simulink model "magnet_field"  (R2023b)
settings: Solver=VariableStepAuto  StartTime=0.0  StopTime=10.0  RelTol=1e-3
values from neighbouring files (symbols this model uses):
  A1 = importdata("igrfSg.txt")    [SAD_project_code.m]
  A2 = importdata("igrfSh.txt")    [SAD_project_code.m]
  n_earth = sqrt(mu_E/a^3)    [SAD_project_code.m]
  timeoflaunch = date2mjd2000(date0)    [SAD_project_code.m]
libraries: simulink_extras x3
settings Model: Creator=edoardonicolucci  LastModifiedBy=edoardonicolucci

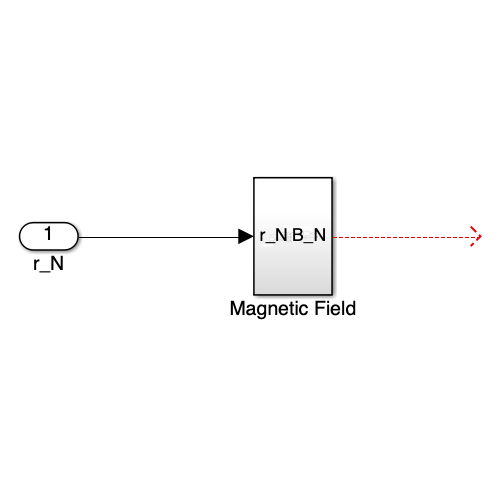
[thumbnail: Simulink's stored preview of the top-level diagram]
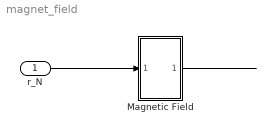
== system magnet_field ==
  r_N : Inport
  Magnetic Field : Subsystem
  wires:
  r_N/1 -> Magnetic Field/1(r_N)
  Magnetic Field/1(B_N) -> ?

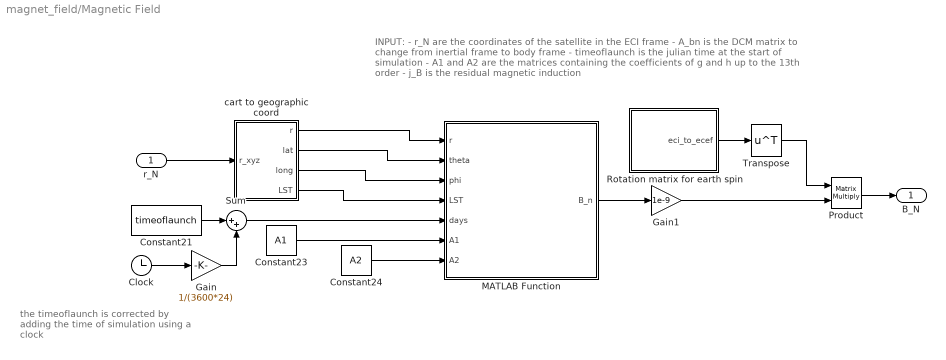
== system magnet_field/Magnetic Field ==
  note: INPUT:
      | - r_N are the coordinates of the satellite in the ECI frame
      | - A_bn is the DCM matrix to change from inertial frame to body frame
      | - timeoflaunch is the julian time at the start of simulation
      | - A1 and A2 are the matrices containing the coefficients of g and h up to the 13th order
      | - j_B is the residual magnetic induction
  note: the timeoflaunch is corrected by adding the time of simulation using a clock
  r_N : Inport
  Clock : Clock
  Constant21 : Constant  Value=timeoflaunch
  Constant23 : Constant  Value=A1
  Constant24 : Constant  Value=A2
  Gain : Gain  Gain=1/(3600*24)
  Gain1 : Gain  Gain=1e-9
  MATLAB Function : MATLAB Function  TreatAsAtomicUnit=on
  Product : Product  Multiplication=Matrix(*)
  Rotation matrix for earth spin : Subsystem
  Sum : Sum  Inputs=|++
  Transpose : Math  Operator=transpose
  cart to geographic coord : Subsystem
  B_N : Outport
  wires:
  Gain/1 -> Sum/2
  Constant23/1 -> MATLAB Function/6(A1)
  Constant24/1 -> MATLAB Function/7(A2)
  Product/1 -> B_N/1
  Constant21/1 -> Sum/1
  MATLAB Function/1(B_n) -> Gain1/1
  cart to geographic coord/4(LST) -> MATLAB Function/4(LST)
  r_N/1 -> cart to geographic coord/1(r_xyz)
  Rotation matrix for earth spin/1(eci_to_ecef) -> Transpose/1
  cart to geographic coord/2(lat) -> MATLAB Function/2(theta)
  Clock/1 -> Gain/1
  Transpose/1 -> Product/1
  cart to geographic coord/3(long) -> MATLAB Function/3(phi)
  Sum/1 -> MATLAB Function/5(days)
  cart to geographic coord/1(r) -> MATLAB Function/1(r)
  Gain1/1 -> Product/2

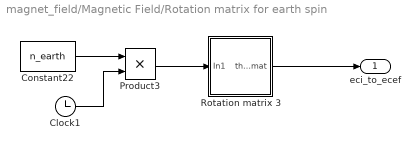
== system magnet_field/Magnetic Field/Rotation matrix for earth spin ==
  Clock1 : Clock
  Constant22 : Constant  Value=n_earth
  Product3 : Product
  Rotation matrix 3 : Subsystem
  eci_to_ecef : Outport
  wires:
  Rotation matrix 3/1(theta_mat) -> eci_to_ecef/1
  Product3/1 -> Rotation matrix 3/1(In1)
  Constant22/1 -> Product3/1
  Clock1/1 -> Product3/2

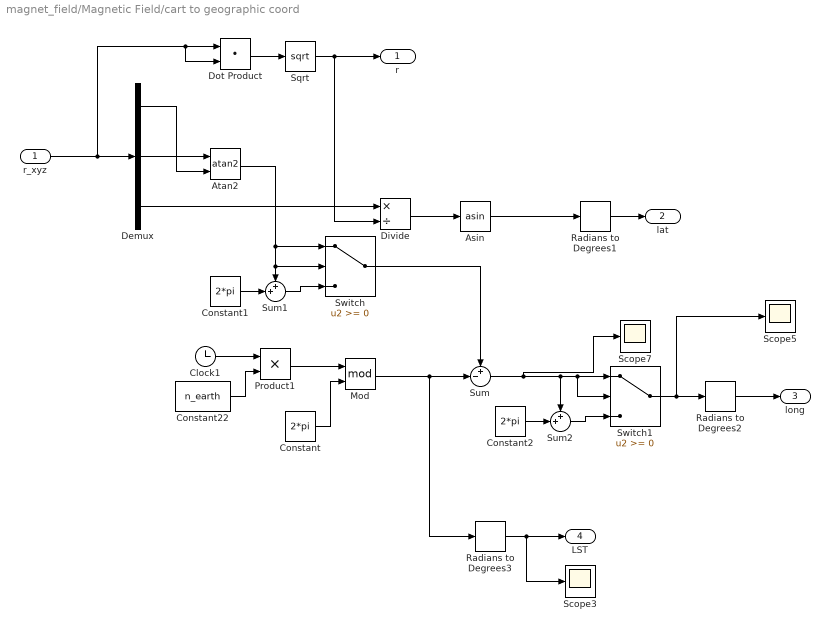
== system magnet_field/Magnetic Field/cart to geographic coord ==
  r_xyz : Inport
  Asin : Trigonometry  Operator=asin
  Atan2 : Trigonometry  Operator=atan2
  Clock1 : Clock
  Constant : Constant  Value=2*pi
  Constant1 : Constant  Value=2*pi
  Constant2 : Constant  Value=2*pi
  Constant22 : Constant  Value=n_earth
  Demux : Demux  Outputs=3
  Divide : Product  Inputs=*/
  Dot Product : DotProduct  OutDataTypeStr=Inherit: Inherit via internal rule
  Mod : Math  Operator=mod
  Product1 : Product
  Radians to Degrees1 : simulink_extras/Transformations/Radians to Degrees
  Radians to Degrees2 : simulink_extras/Transformations/Radians to Degrees
  Radians to Degrees3 : simulink_extras/Transformations/Radians to Degrees
  Scope3 : Scope
  Scope5 : Scope
  Scope7 : Scope
  Sqrt : Sqrt
  Sum : Sum  Inputs=+-|
  Sum1 : Sum  Inputs=++|
  Sum2 : Sum  Inputs=++|
  Switch : Switch  SaturateOnIntegerOverflow=off  InputSameDT=off
  Switch1 : Switch  SaturateOnIntegerOverflow=off  InputSameDT=off
  r : Outport
  lat : Outport  Port=2
  long : Outport  Port=3
  LST : Outport  Port=4
  wires:
  r_xyz/1 -> Dot Product/2, Dot Product/1, Demux/1
  Asin/1 -> Radians to Degrees1/1
  Dot Product/1 -> Sqrt/1
  Sqrt/1 -> r/1, Divide/2
  Demux/3 -> Divide/1
  Divide/1 -> Asin/1
  Demux/2 -> Atan2/1
  Demux/1 -> Atan2/2
  Constant22/1 -> Product1/2
  Clock1/1 -> Product1/1
  Sum/1 -> Scope7/1, Sum2/1, Switch1/2, Switch1/1
  Radians to Degrees3/1 -> Scope3/1, LST/1
  Mod/1 -> Radians to Degrees3/1, Sum/2
  Constant/1 -> Mod/2
  Atan2/1 -> Switch/1, Sum1/1, Switch/2
  Sum1/1 -> Switch/3
  Constant1/1 -> Sum1/2
  Sum2/1 -> Switch1/3
  Constant2/1 -> Sum2/2
  Switch1/1 -> Scope5/1, Radians to Degrees2/1
  Switch/1 -> Sum/1
  Radians to Degrees1/1 -> lat/1
  Radians to Degrees2/1 -> long/1
  Product1/1 -> Mod/1

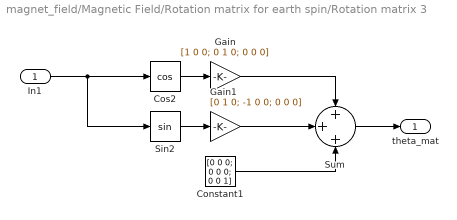
== system magnet_field/Magnetic Field/Rotation matrix for earth spin/Rotation matrix 3 ==
  In1 : Inport
  Constant1 : Constant  Value=[0 0 0; 0 0 0; 0 0 1]
  Cos2 : Trigonometry  Operator=cos
  Gain : Gain  Gain=[1 0 0; 0 1 0; 0 0 0]
  Gain1 : Gain  Gain=[0 1 0; -1 0 0; 0 0 0]
  Sin2 : Trigonometry
  Sum : Sum  Inputs=+++
  theta_mat : Outport
  wires:
  Cos2/1 -> Gain/1
  Gain/1 -> Sum/1
  In1/1 -> Sin2/1, Cos2/1
  Sin2/1 -> Gain1/1
  Sum/1 -> theta_mat/1
  Gain1/1 -> Sum/2
  Constant1/1 -> Sum/3

== matlab function magnet_field/Magnetic Field/MATLAB Function ==
  data: r input; B_n output; theta input; phi input; LST input; days input; A1 input; A2 input
function B_n = magnetic_field_model(r, theta, phi, LST, days, A1, A2)
%   mjd2000[1]  Date in MJD 2000. MJD2000 is defined as the number of days
%               since 01-01-2000, 12:00 noon.

% Inputs
% r         Geocentric radius
% theta     Latitude measured in degrees positive from equator  
% phi       Longitude measured in degrees positive east from Greenwich
% days      Decimal days since January 1, 2020
%
% Outputs - magnetic field strength in local tangential coordinates
% Br    B in radial direction
% Bt    B in theta direction
% Bp    B in phi direction
[Br,Bt,Bp] = magnet(r,theta,phi,days, 1, A1, A2);
%[Br, Bt, Bp] = igrf(gh, theta, phi, r, 'geocentric');



% Inputs
% Br    B in radial direction
% Bt    B in theta direction
% Bp    B in phi direction
% LST   Local sidereal time of location (in degrees)(right ascension)
% lat   Latitude measured positive north from equator (in degrees), it is
%       the same as the local declination
%
% Outputs
% Bx    B in x-direction  | Magnetic field strength (B)
% By    B in y-direction  | in geocentric inertial coordinates
% Bz    B in z-direction  |
[Bx,By,Bz] = msph2inert(Br,Bt,Bp, phi, theta);

B_n = [Bx,By,Bz]';
